simulink model "lane_stop_sl"  (R2019a)
settings: Solver=FixedStepDiscrete  StartTime=0.0  StopTime=inf  FixedStep=0.1  RelTol=1e-3  EnableMultiTasking=on
model workspace (MAT data in the model file):
  SL_ROS_VariableLengthArrays_MaxSizes.CommonInfo.ArrayTruncateAction = 'EmitWarning'
  SL_ROS_VariableLengthArrays_MaxSizes.MsgTypeMap = containers.Map
  SL_ROS_VariableLengthArrays_MaxSizes.MsgTypeMap.serialization.keys = {'autoware_msgs/Lane', 'autoware_msgs/LaneArray', 'autoware_msgs/lane'}
  SL_ROS_VariableLengthArrays_MaxSizes.MsgTypeMap.serialization.values{1}.PropertyName = 'Waypoints'
  SL_ROS_VariableLengthArrays_MaxSizes.MsgTypeMap.serialization.values{1}.DataType = 'autoware_msgs/Waypoint'
  SL_ROS_VariableLengthArrays_MaxSizes.MsgTypeMap.serialization.values{1}.MaxLength = 100
  SL_ROS_VariableLengthArrays_MaxSizes.MsgTypeMap.serialization.values{2}.PropertyName = 'Lanes'
  SL_ROS_VariableLengthArrays_MaxSizes.MsgTypeMap.serialization.values{2}.DataType = 'autoware_msgs/lane'
  SL_ROS_VariableLengthArrays_MaxSizes.MsgTypeMap.serialization.values{2}.MaxLength = 100
  SL_ROS_VariableLengthArrays_MaxSizes.MsgTypeMap.serialization.values{3}.PropertyName = 'Waypoints'
  SL_ROS_VariableLengthArrays_MaxSizes.MsgTypeMap.serialization.values{3}.DataType = 'autoware_msgs/waypoint'
  SL_ROS_VariableLengthArrays_MaxSizes.MsgTypeMap.serialization.values{3}.MaxLength = 100
  SL_ROS_VariableLengthArrays_MaxSizes.MsgTypeMap.serialization.uniformity = 0
  SL_ROS_VariableLengthArrays_MaxSizes.MsgTypeMap.serialization.keyType = 'char'
  SL_ROS_VariableLengthArrays_MaxSizes.MsgTypeMap.serialization.valueType = 'any'
libraries: robotlib x6
settings Model: Creator=tkikawad  LastModifiedBy=root
settings DataIOCC: ReturnWorkspaceOutputs=off
settings DebuggingCC: ArithmeticOperatorsInVariantConditions=warning
settings SFSimCC: SimUseLocalCustomCode=off
settings RTWCC: RTWUseLocalCustomCode=off
settings CodeAppCC: StateflowObjectComments=on

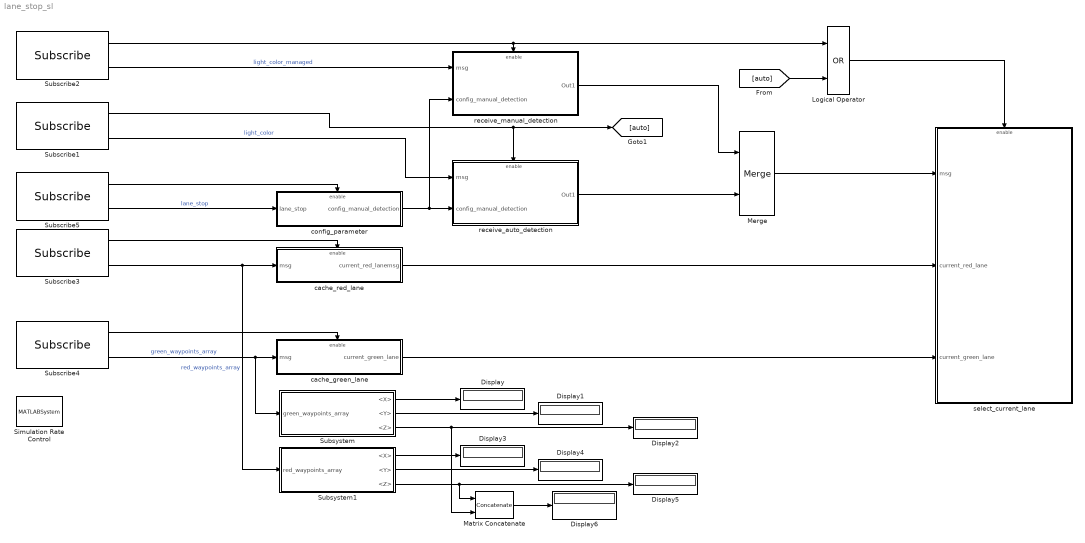
== system lane_stop_sl ==
  Display{,1..6} (7 alike) : Display
  Logical Operator : Logic  Operator=OR  AllPortsSameDT=off  OutDataTypeStr=boolean
  Matrix Concatenate : Concatenate  Mode=Multidimensional array  ConcatenateDimension=2
  Merge : Merge
  Simulation Rate Control : MATLABSystem  System=ExampleHelperSimulationRateControl  SampleTime=0.1
      mask Type: ExampleHelperSimulationRateControl
      mask Display: disp('Rate Control');
  Subscribe1 : robotlib/Subscribe  topicSource=Specify your own  topic=/light_color  messageType=autoware_msgs/TrafficLight  sampleTime=-1  messageQueueLength=1
      settings: SourceProductBaseCode=RO
  Subscribe2 : robotlib/Subscribe  topicSource=Specify your own  topic=/light_color_managed  messageType=autoware_msgs/TrafficLight  sampleTime=-1  messageQueueLength=1
      settings: SourceProductBaseCode=RO
  Subscribe3 : robotlib/Subscribe  topicSource=Specify your own  topic=/red_waypoints_array  messageType=autoware_msgs/LaneArray  sampleTime=-1  messageQueueLength=1
      settings: SourceProductBaseCode=RO
  Subscribe4 : robotlib/Subscribe  topicSource=Specify your own  topic=/green_waypoints_array  messageType=autoware_msgs/LaneArray  sampleTime=-1  messageQueueLength=1
      settings: SourceProductBaseCode=RO
  Subscribe5 : robotlib/Subscribe  topicSource=Specify your own  topic=/config/lane_stop  messageType=autoware_config_msgs/ConfigLaneStop  sampleTime=-1  messageQueueLength=1
      settings: SourceProductBaseCode=RO
  Subsystem : Subsystem
  Subsystem1 : Subsystem
  cache_green_lane : Subsystem
  cache_red_lane : Subsystem
  config_parameter : Subsystem
  receive_auto_detection : Subsystem
  receive_manual_detection : Subsystem
  select_current_lane : Subsystem
  wires:
  Subscribe1/1 -> receive_auto_detection/Enable, [auto]
  Subscribe3/1 -> cache_red_lane/Enable
  Subscribe5/1 -> config_parameter/Enable
  Subscribe3/2 -> cache_red_lane/1(msg), Subsystem1/1(red_waypoints_array)  "red_waypoints_array"
  Subsystem/1(<X>) -> Display/1
  Subsystem/2(<Y>) -> Display1/1
  Subsystem/3(<Z>) -> Matrix Concatenate/2, Display2/1
  Subsystem1/3(<Z>) -> Matrix Concatenate/1, Display5/1
  Subsystem1/2(<Y>) -> Display4/1
  Subsystem1/1(<X>) -> Display3/1
  Matrix Concatenate/1 -> Display6/1
  Subscribe5/2 -> config_parameter/1(lane_stop)  "lane_stop"
  config_parameter/1(config_manual_detection) -> receive_manual_detection/2(config_manual_detection), receive_auto_detection/2(config_manual_detection)
  Subscribe1/2 -> receive_auto_detection/1(msg)  "light_color"
  Subscribe2/2 -> receive_manual_detection/1(msg)  "light_color_managed"
  Subscribe2/1 -> Logical Operator/1, receive_manual_detection/Enable
  receive_manual_detection/1(Out1) -> Merge/1
  receive_auto_detection/1(Out1) -> Merge/2
  Merge/1 -> select_current_lane/1(msg)
  cache_red_lane/1(current_red_lanemsg) -> select_current_lane/2(current_red_lane)
  Subscribe4/2 -> cache_green_lane/1(msg), Subsystem/1(green_waypoints_array)  "green_waypoints_array"
  Subscribe4/1 -> cache_green_lane/Enable
  cache_green_lane/1(current_green_lane) -> select_current_lane/3(current_green_lane)
  [auto] -> Logical Operator/2
  Logical Operator/1 -> select_current_lane/Enable

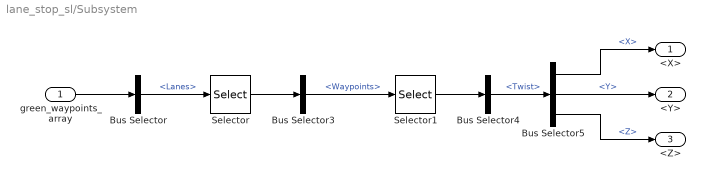
== system lane_stop_sl/Subsystem ==
  green_waypoints_array : Inport
  Bus Selector : BusSelector  OutputSignals=Lanes
  Bus Selector3 : BusSelector  OutputSignals=Waypoints
  Bus Selector4 : BusSelector  OutputSignals=Twist
  Bus Selector5 : BusSelector  OutputSignals=Twist.Linear.X,Twist.Linear.Y,Twist.Linear.Z
  Selector : Selector  InputPortWidth=100  IndexOptions=Index vector (dialog)  Indices=1  OutputSizes=1
  Selector1 : Selector  InputPortWidth=100  IndexOptions=Index vector (dialog)  Indices=80  OutputSizes=1
  <X> : Outport
  <Y> : Outport  Port=2
  <Z> : Outport  Port=3
  wires:
  Selector/1 -> Bus Selector3/1
  Bus Selector/1 -> Selector/1  "<Lanes>"
  Bus Selector5/1 -> <X>/1  "<X>"
  green_waypoints_array/1 -> Bus Selector/1
  Bus Selector4/1 -> Bus Selector5/1  "<Twist>"
  Bus Selector5/3 -> <Z>/1  "<Z>"
  Bus Selector5/2 -> <Y>/1  "<Y>"
  Selector1/1 -> Bus Selector4/1
  Bus Selector3/1 -> Selector1/1  "<Waypoints>"

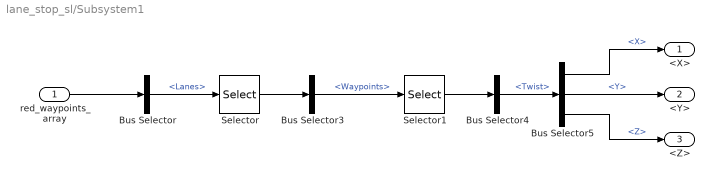
== system lane_stop_sl/Subsystem1 ==
  red_waypoints_array : Inport
  Bus Selector : BusSelector  OutputSignals=Lanes
  Bus Selector3 : BusSelector  OutputSignals=Waypoints
  Bus Selector4 : BusSelector  OutputSignals=Twist
  Bus Selector5 : BusSelector  OutputSignals=Twist.Linear.X,Twist.Linear.Y,Twist.Linear.Z
  Selector : Selector  InputPortWidth=100  IndexOptions=Index vector (dialog)  Indices=1  OutputSizes=1
  Selector1 : Selector  InputPortWidth=100  IndexOptions=Index vector (dialog)  Indices=1  OutputSizes=1
  <X> : Outport
  <Y> : Outport  Port=2
  <Z> : Outport  Port=3
  wires:
  Bus Selector3/1 -> Selector1/1  "<Waypoints>"
  Selector1/1 -> Bus Selector4/1
  Bus Selector5/2 -> <Y>/1  "<Y>"
  Bus Selector5/3 -> <Z>/1  "<Z>"
  Bus Selector4/1 -> Bus Selector5/1  "<Twist>"
  red_waypoints_array/1 -> Bus Selector/1
  Bus Selector5/1 -> <X>/1  "<X>"
  Bus Selector/1 -> Selector/1  "<Lanes>"
  Selector/1 -> Bus Selector3/1

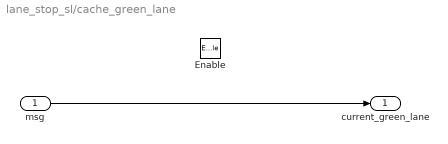
== system lane_stop_sl/cache_green_lane ==
  msg : Inport
  Enable : EnablePort
  current_green_lane : Outport
  wires:
  msg/1 -> current_green_lane/1

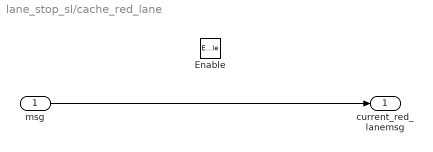
== system lane_stop_sl/cache_red_lane ==
  msg : Inport
  Enable : EnablePort
  current_red_lanemsg : Outport
  wires:
  msg/1 -> current_red_lanemsg/1

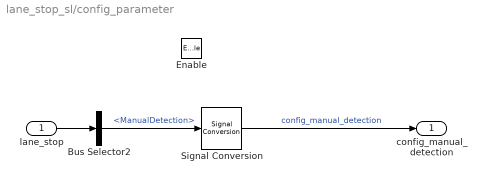
== system lane_stop_sl/config_parameter ==
  lane_stop : Inport
  Enable : EnablePort
  Bus Selector2 : BusSelector  OutputSignals=ManualDetection
  Signal Conversion : SignalConversion  OverrideOpt=off
  config_manual_detection : Outport
  wires:
  Bus Selector2/1 -> Signal Conversion/1  "<ManualDetection>"
  lane_stop/1 -> Bus Selector2/1
  Signal Conversion/1 -> config_manual_detection/1  "config_manual_detection"

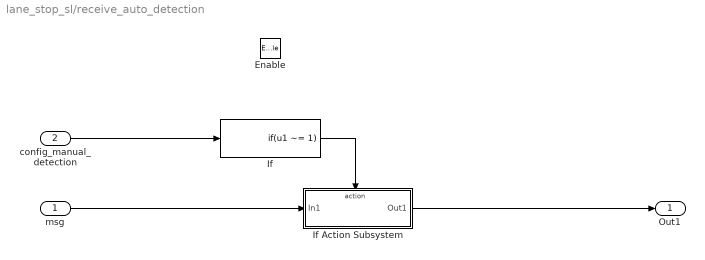
== system lane_stop_sl/receive_auto_detection ==
  msg : Inport
  config_manual_detection : Inport  Port=2
  Enable : EnablePort
  If : If  IfExpression=u1 ~= 1  ShowElse=off
  If Action Subsystem : Subsystem  TreatAsAtomicUnit=on
  Out1 : Outport
  wires:
  config_manual_detection/1 -> If/1
  msg/1 -> If Action Subsystem/1(In1)
  If/1 -> If Action Subsystem/Action
  If Action Subsystem/1(Out1) -> Out1/1

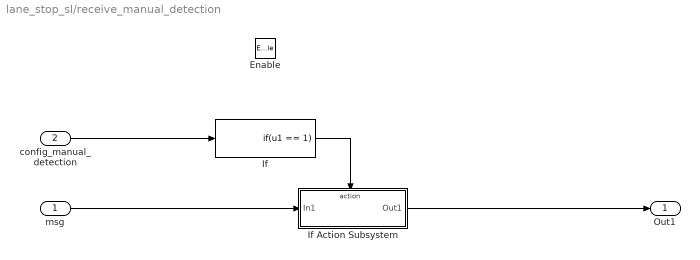
== system lane_stop_sl/receive_manual_detection ==
  msg : Inport
  config_manual_detection : Inport  Port=2
  Enable : EnablePort
  If : If  IfExpression=u1 == 1  ShowElse=off
  If Action Subsystem : Subsystem  TreatAsAtomicUnit=on
  Out1 : Outport
  wires:
  If Action Subsystem/1(Out1) -> Out1/1
  If/1 -> If Action Subsystem/Action
  msg/1 -> If Action Subsystem/1(In1)
  config_manual_detection/1 -> If/1

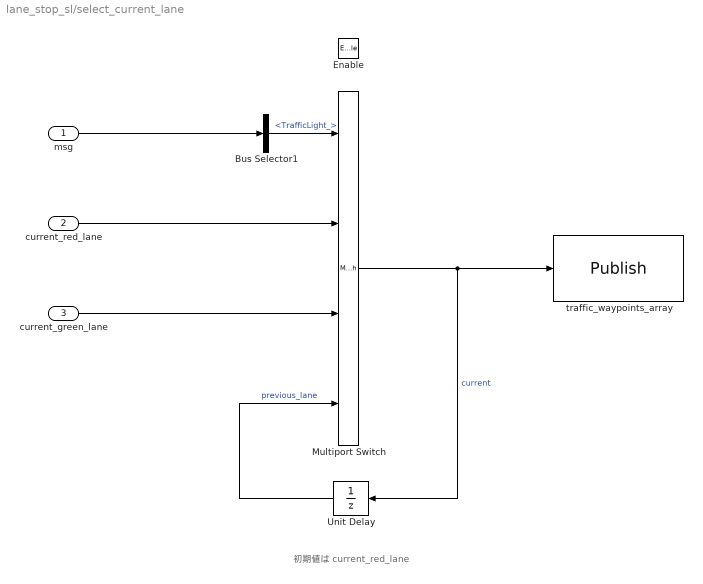
== system lane_stop_sl/select_current_lane ==
  note: 初期値は current_red_lane
  msg : Inport
  current_red_lane : Inport  Port=2
  current_green_lane : Inport  Port=3
  Enable : EnablePort
  Bus Selector1 : BusSelector  OutputSignals=TrafficLight_
  Multiport Switch : MultiPortSwitch  DataPortOrder=Zero-based contiguous  DiagnosticForDefault=None  zeroidx=on
  Unit Delay : UnitDelay  SampleTime=-1  HasFrameUpgradeWarning=on
  traffic_waypoints_array : robotlib/Publish  topicSource=Specify your own  topic=/traffic_waypoints_array  messageType=autoware_msgs/LaneArray  messageQueueLength=1
      settings: SourceProductBaseCode=RO
  wires:
  msg/1 -> Bus Selector1/1
  Bus Selector1/1 -> Multiport Switch/1  "<TrafficLight_>"
  Multiport Switch/1 -> traffic_waypoints_array/1, Unit Delay/1  "current"
  current_green_lane/1 -> Multiport Switch/3
  current_red_lane/1 -> Multiport Switch/2
  Unit Delay/1 -> Multiport Switch/4  "previous_lane"

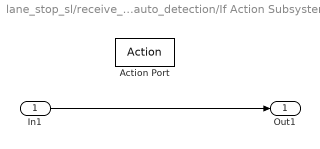
== system lane_stop_sl/receive_auto_detection/If Action Subsystem ==
  In1 : Inport
  Action Port : ActionPort  ActionPortLabel=if(u1 ~= 1)
  Out1 : Outport
  wires:
  In1/1 -> Out1/1

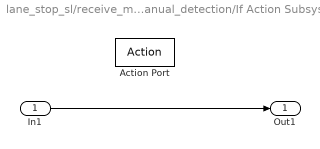
== system lane_stop_sl/receive_manual_detection/If Action Subsystem ==
  In1 : Inport
  Action Port : ActionPort  ActionPortLabel=if(u1 == 1)
  Out1 : Outport
  wires:
  In1/1 -> Out1/1
